simulink model "Android_interface"  (R2017a)
settings: Solver=FixedStepDiscrete  StartTime=0.0  StopTime=inf  FixedStep=0.002  RelTol=1e-3
libraries: androidlib x10
settings Model: SimulationMode=external  ExtModeTrigDuration=10000  Creator=gjaniak  LastModifiedBy=gjaniak
settings SolverCC: PositivePriorityOrder=on
settings OptimizationCC: PassReuseOutputArgsThreshold=0  MaxStackSize=64
settings DebuggingCC: ParameterTunabilityLossMsg=error
settings HardwareCC: ProdBitPerPointer=32  ProdBitPerSizeT=32  ProdBitPerPtrDiffT=32  ProdLargestAtomicInteger=Long  ProdLargestAtomicFloat=Double  ProdWordSize=32  ProdHWDeviceType=ARM Compatible->ARM Cortex  UseEmbeddedCoderFeatures=off
settings RTWCC: SystemTargetFile=ert.tlc  HardwareBoard=Android Device  TLCOptions="-aInlineSetEventsForThisBaseRateFcn=TLC_FALSE -aSuppressMultiTaskScheduler=TLC_FALSE  -aRateBasedStepFcn=0"  TemplateMakefile=ert_default_tmf  Description=Embedded Coder  GenerateReport=on  Toolchain=Android SDK/NDK Tools  LaunchReport=on
settings CodeAppCC: ForceParamTrailComments=on  OperatorAnnotations=on  MATLABSourceComments=on
settings ERTTargetCC: MultiwordLength=2048  ERTCustomFileBanners=off  SupportContinuousTime=on  SupportNonInlinedSFcns=on  RemoveResetFunc=off  ModelStepFunctionPrototypeControlCompliant=off

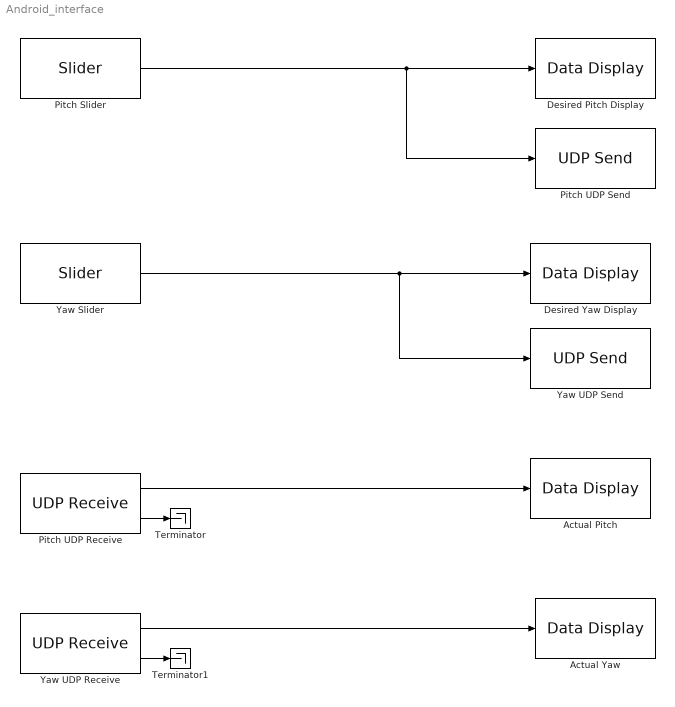
== system Android_interface ==
  Actual Pitch : androidlib/Data Display  DataDisplayId=Android_interface_Actual_Pitch  Format=Float  Precision=6  SimulateUsing=Code generation  blockPlatform=Android
      settings: SourceProductName=Simulink Support Package for Android Devices  SourceProductBaseCode=ANDROID
  Actual Yaw : androidlib/Data Display  DataDisplayId=Android_interface_Actual_Yaw  Format=Float  Precision=6  SimulateUsing=Code generation  blockPlatform=Android
      settings: SourceProductName=Simulink Support Package for Android Devices  SourceProductBaseCode=ANDROID
  Desired Pitch Display : androidlib/Data Display  DataDisplayId=Android_interface_Desired_Pitch_Display  Format=Float  Precision=6  SimulateUsing=Code generation  blockPlatform=Android
      settings: SourceProductName=Simulink Support Package for Android Devices  SourceProductBaseCode=ANDROID
  Desired Yaw Display : androidlib/Data Display  DataDisplayId=Android_interface_Desired_Yaw_Display  Format=Float  Precision=6  SimulateUsing=Code generation  blockPlatform=Android
      settings: SourceProductName=Simulink Support Package for Android Devices  SourceProductBaseCode=ANDROID
  Pitch Slider : androidlib/Slider  Min=-80  Value=0  Max=80  Resolution=1  SliderId=Android_interface_Pitch_Slider  SampleTime=0.1  BlockPlatform=Android
      settings: SourceProductName=Simulink Support Package for Android Devices  SourceProductBaseCode=ANDROID
  Pitch UDP Receive : androidlib/UDP Receive  localURL='0.0.0.0'  localPort=26002  remoteURL='0.0.0.0'  remotePort=-1  recvBufferSize=8192  signalDatatype=double  dims=1  isVarSize=off  showBlockingTime=off  blockingTime=0  sampletime=0.01  blockPlatform=Android
      settings: SourceProductName=Simulink Support Package for Android Devices  SourceProductBaseCode=ANDROID
  Pitch UDP Send : androidlib/UDP Send  remoteURL='192.168.1.20'  remotePort=26000  localURL='0.0.0.0'  localPortSource=Automatically determine  localPort=-1  sampletime=-1  blockPlatform=Android  separateLengthPort=0
      settings: SourceProductName=Simulink Support Package for Android Devices  SourceProductBaseCode=ANDROID
  Terminator : Terminator
  Terminator1 : Terminator
  Yaw Slider : androidlib/Slider  Min=-180  Value=0  Max=180  Resolution=1  SliderId=Android_interface_Yaw_Slider  SampleTime=0.1  BlockPlatform=Android
      settings: SourceProductName=Simulink Support Package for Android Devices  SourceProductBaseCode=ANDROID
  Yaw UDP Receive : androidlib/UDP Receive  localURL='0.0.0.0'  localPort=26003  remoteURL='0.0.0.0'  remotePort=-1  recvBufferSize=8192  signalDatatype=double  dims=1  isVarSize=off  showBlockingTime=off  blockingTime=0  sampletime=0.01  blockPlatform=Android
      settings: SourceProductName=Simulink Support Package for Android Devices  SourceProductBaseCode=ANDROID
  Yaw UDP Send : androidlib/UDP Send  remoteURL='192.168.1.20'  remotePort=26001  localURL='0.0.0.0'  localPortSource=Automatically determine  localPort=-1  sampletime=-1  blockPlatform=Android  separateLengthPort=0
      settings: SourceProductName=Simulink Support Package for Android Devices  SourceProductBaseCode=ANDROID
  wires:
  Yaw UDP Receive/1 -> Actual Yaw/1
  Pitch UDP Receive/1 -> Actual Pitch/1
  Yaw Slider/1 -> Yaw UDP Send/1, Desired Yaw Display/1
  Pitch Slider/1 -> Pitch UDP Send/1, Desired Pitch Display/1
  Pitch UDP Receive/2 -> Terminator/1
  Yaw UDP Receive/2 -> Terminator1/1
